simulink model "Senalizacion"  (R2023b)
settings: Solver=VariableStepAuto  StartTime=0.0  StopTime=10.0  RelTol=1e-3
libraries: arduinolib x5, simulink x2
settings Model: Creator=chris  LastModifiedBy=chris

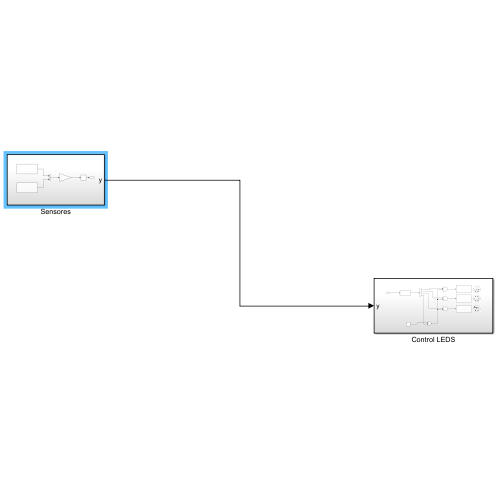
[thumbnail: Simulink's stored preview of the top-level diagram]
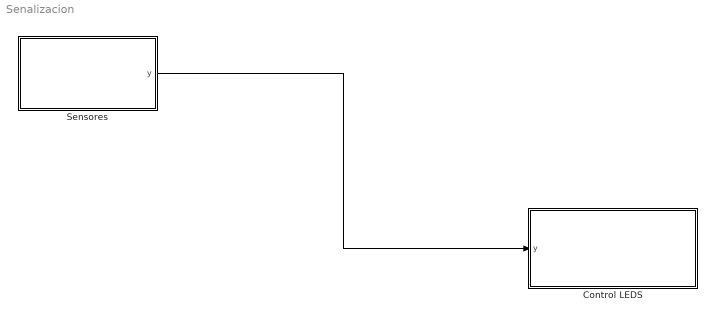
== system Senalizacion ==
  Control LEDS : Subsystem
  Sensores : Subsystem
  wires:
  Sensores/1(y) -> Control LEDS/1(y)

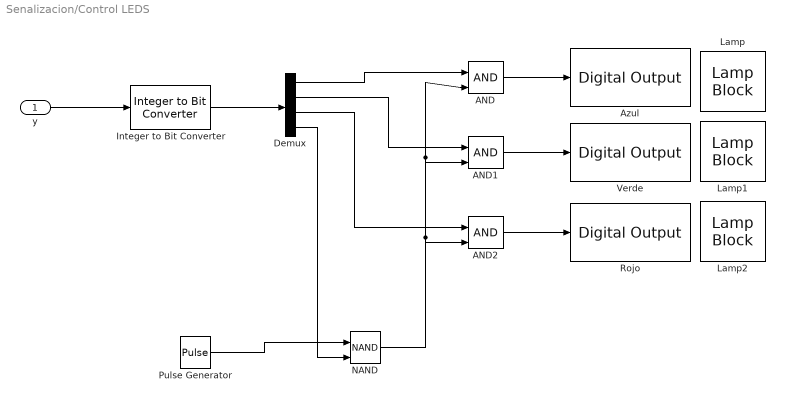
== system Senalizacion/Control LEDS ==
  y : Inport
  AND : Logic  IconShape=distinctive  AllPortsSameDT=off  OutDataTypeStr=boolean
  AND1 : Logic  IconShape=distinctive  AllPortsSameDT=off  OutDataTypeStr=boolean
  AND2 : Logic  IconShape=distinctive  AllPortsSameDT=off  OutDataTypeStr=boolean
  Azul : arduinolib/Digital Output  pinNumber=33  Direction=output  blockPlatform=arduino
  Demux : Demux
  Integer to Bit Converter : simulink/Logic and Bit Operations/Integer to Bit Converter  nbits=3  signedInputValues=Unsigned  bitOrder=MSB first  outDtype=Inherit via internal rule
  Lamp : LampBlock  LabelPosition=Hide
  Lamp1 : LampBlock  LabelPosition=Hide
  Lamp2 : LampBlock  LabelPosition=Hide
  NAND : Logic  Operator=NAND  IconShape=distinctive  AllPortsSameDT=off  OutDataTypeStr=boolean
  Pulse Generator : DiscretePulseGenerator  PulseType=Time based  Period=10  PulseWidth=5
  Rojo : arduinolib/Digital Output  pinNumber=46  Direction=output  blockPlatform=arduino
  Verde : arduinolib/Digital Output  pinNumber=31  Direction=output  blockPlatform=arduino
  wires:
  AND2/1 -> Rojo/1
  Demux/3 -> AND2/1
  Demux/1 -> AND/1
  NAND/1 -> AND2/2, AND1/2, AND/2
  Pulse Generator/1 -> NAND/1
  y/1 -> Integer to Bit Converter/1
  AND1/1 -> Verde/1
  Integer to Bit Converter/1 -> Demux/1
  AND/1 -> Azul/1
  Demux/4 -> NAND/2
  Demux/2 -> AND1/1

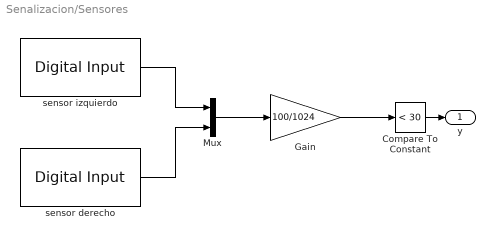
== system Senalizacion/Sensores ==
  Compare To Constant : simulink/Logic and Bit Operations/Compare To Constant  relop=<  const=30  OutDataTypeStr=boolean
  Gain : Gain  Gain=100/1024
  Mux : Mux  Inputs=2
  sensor derecho : arduinolib/Digital Input  pinNumber=8  mode=Default  Direction=input  SampleTime=0.1  blockPlatform=arduino
  sensor izquierdo : arduinolib/Digital Input  pinNumber=8  mode=Default  Direction=input  SampleTime=0.1  blockPlatform=arduino
  y : Outport
  wires:
  Compare To Constant/1 -> y/1
  sensor derecho/1 -> Mux/2
  Gain/1 -> Compare To Constant/1
  Mux/1 -> Gain/1
  sensor izquierdo/1 -> Mux/1
